simulink model "Pacemaker_A2_10_pushButton_bonus"  (R2020a)
settings: Solver=FixedStepAuto  StartTime=0.0  StopTime=10.0  FixedStep=1e-3  RelTol=1e-3  EnableMultiTasking=on
undefined symbols (not defined in the file): A0, A1, D0, D1, D10, D11, D12, D13, D2, D3, D4, D5, D6, D7, D8, D9, PTA0, PTA1, PTA2, PTB2, PTB23, PTB3, PTB9, PTC16, PTC17, PTC2, PTC3, PTC4, PTD0, PTD1, PTD2, PTD3
libraries: frdmk64flib x30, etargetslib x4
settings Model: ExtModeTrigDuration=5  Creator=forre  LastModifiedBy=forre
settings OptimizationCC: EnhancedBackFolding=on  PassReuseOutputArgsAs=Individual arguments  ZeroExternalMemoryAtStartup=off  ZeroInternalMemoryAtStartup=off  MaxStackSize=64  OptimizeBlockOrder=speed  DifferentSizesBufferReuse=on  OptimizationCustomize=off  EfficientTunableParamExpr=on
settings DebuggingCC: ParameterTunabilityLossMsg=error
settings HardwareCC: ProdBitPerPointer=32  ProdBitPerSizeT=32  ProdBitPerPtrDiffT=32  ProdLargestAtomicInteger=Long  ProdLargestAtomicFloat=Double  ProdWordSize=32  ProdHWDeviceType=ARM Compatible->ARM Cortex
settings SFSimCC: MATLABDynamicMemAlloc=off
settings RTWCC: SystemTargetFile=ert.tlc  HardwareBoard=NXP FRDM-K64F  TemplateMakefile=ert_default_tmf  Toolchain=GNU Tools for ARM Embedded Processors
settings CodeAppCC: ForceParamTrailComments=on  IgnoreCustomStorageClasses=off  OperatorAnnotations=on  SimulinkDataObjDesc=on  SFDataObjDesc=on  InsertBlockDesc=on

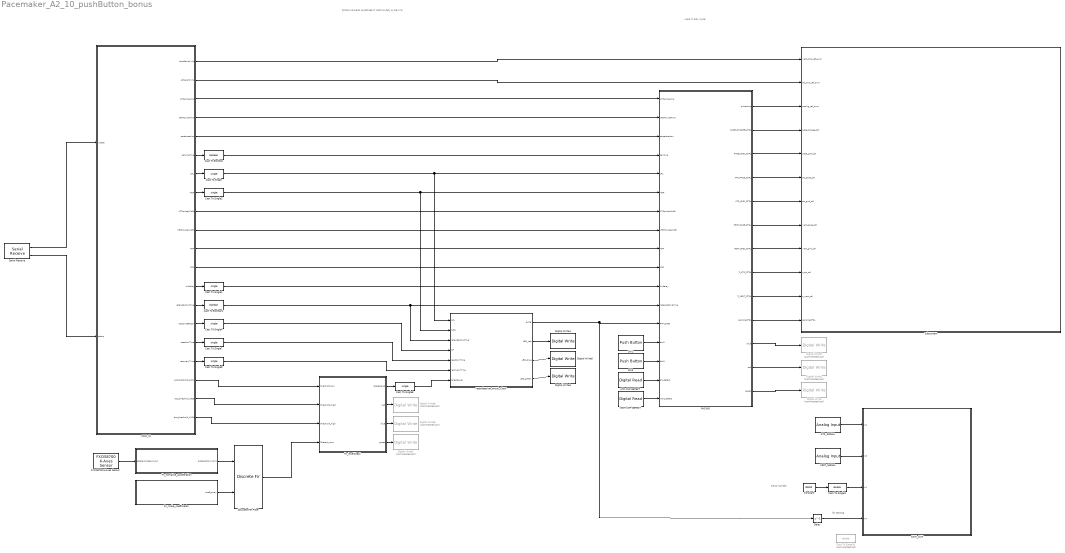
== system Pacemaker_A2_10_pushButton_bonus ==
  note: for testing
  note: serial number
  note: Python converts amplitude in Volts to duty cycle in %
  note: input = duty cycle
  ATR CMP DETECT : frdmk64flib/Digital Read  Whichpin=PTC16 (D0)  SampleTime=-1
  ATR_SIGNAL : frdmk64flib/Analog Input  Whichpin=PTB2 (A0)  SampleTime=0.01
  COM_IN : Stateflow chart  TreatAsAtomicUnit=on
      settings: PortSchema="{\"entries\":[{\"content\":{\"sides\":[{\"content\":{\"connectorIds\":[\"In1\",\"In2\"]},\"type\":\"ConnectorPlacement.EquallySpacedRectSide\",\"uuid\":\"708f6c47-59ba-4c62-823e-aceb534f7d4e\"},{\"content\":{\"connectorIds\":[\"Out1\",\"Out3\",\"Out2\",\"Out4\",\"Out5\",\"Out6\",\"Out7\",\"Out8\",\"Out9\",\"Out10\",\"Out11\",\"Out12\",\"Out13\",\"Out14\",\"Out15\",\"Out16\",\"Out17\",\"Out18\",\"Out19\",\"Out20\"],\"side\":\"RIGHT\"},\"type\":\"ConnectorPlacement.EquallySpacedRectSide\",\"uuid\":\"fc195095-7643-467f-bfab-06db9c9b4f5e\"},{\"content\":{\"connectorIds\":[],\"side\":\"TOP\"},\"type\":\"ConnectorPlacement.EquallySpacedRectSide\",\"uuid\":\"2b9dc66d-b3fc-4626-8ab6-5dc1815dc2f6\"}]},\"type\":\"ConnectorPlacement.EquallySpacedConnector\",\"uuid\":\"ad24e883-72a0-4c10-9901-797c84f459ab\"}],\"packageUris\":[\"http://schema.mathworks.com/mf0/Connector/19700101\"],\"version\":\"1.0\"}"
  COM_OUT : Subsystem
  Cast To Boolean : DataTypeConversion  OutDataTypeStr=boolean
  Cast To Boolean1 : DataTypeConversion  OutDataTypeStr=boolean
  Cast To Single{,1..2,4,7..9} (7 alike) : DataTypeConversion  OutDataTypeStr=single
  Cast To Single10 : DataTypeConversion  Commented=on  OutDataTypeStr=double
  Cast To Single3 : DataTypeConversion  OutDataTypeStr=double
  Constant : Constant  Value=92020
  Delay : Delay  DelayLength=1
  Digital Write : frdmk64flib/Digital Write  Commented=on  Whichpin=GREEN_LED
  Digital Write1 : frdmk64flib/Digital Write  Commented=on  Whichpin=RED_LED
  Digital Write2 : frdmk64flib/Digital Write  Commented=on  Whichpin=GREEN_LED
  Digital Write3 : frdmk64flib/Digital Write  Whichpin=GREEN_LED
  Digital Write4 : frdmk64flib/Digital Write  Whichpin=RED_LED
  Digital Write5 : frdmk64flib/Digital Write  Whichpin=BLUE_LED
  Digital Write6 : frdmk64flib/Digital Write  Commented=on  Whichpin=RED_LED
  Digital Write7 : frdmk64flib/Digital Write  Commented=on  Whichpin=BLUE_LED
  Digital Write8 : frdmk64flib/Digital Write  Commented=on  Whichpin=BLUE_LED
  Discrete FIR Filter : DiscreteFir  CoefSource=Input port  Coefficients=[0.05, 0.05, 0.05, 0.05, 0.05, 0.05, 0.05, 0.05, 0.05, 0.05, 0.05, 0.05, 0.05, 0.05, 0.05, 0.05, 0.05, 0.05, 0.05, 0.05]  SampleTime=0.01
      settings: InputPortMap=u0,u1
  FXOS8700 6-Axes Sensor : frdmk64flib/FXOS8700 6-Axes Sensor  Activesensor=Accelerometer only  ODR=800Hz  HybridODR=400Hz  Accelfullrange=-4g to +4g  SampleTime=-1
  Fn_levelCheck : MATLAB Function  TreatAsAtomicUnit=on
  Fn_make_coefficients : MATLAB Function  TreatAsAtomicUnit=on
  Fn_nomalize_acceleration : MATLAB Function  TreatAsAtomicUnit=on
  PACING : Stateflow chart  TreatAsAtomicUnit=on
  SW2 : frdmk64flib/Push Button  Whichswitch=SW2  SampleTime1=-1
  SW3 : frdmk64flib/Push Button  Whichswitch=SW3  SampleTime1=-1
  Serial Receive : frdmk64flib/Serial Receive  SCIModule=0  Baudrate=uint32(9600)  Parity=None  StopBits=1  HardwareFlowControl=None  ByteOrder=LittleEndian  DataType=uint8  DataLength=57  BlockingMode=off  OutputStatus=on  SampleTime=-1
  Subsystem : Subsystem
  VENT CMP DETECT : frdmk64flib/Digital Read  Whichpin=PTC17 (D1)  SampleTime=-1
  VENT_SIGNAL : frdmk64flib/Analog Input  Whichpin=PTB3 (A1)  SampleTime=0.01
  rateAdaptiveControl_Chart : Stateflow chart  TreatAsAtomicUnit=on
  wires:
  SW2/1 -> PACING/14(btn2)
  PACING/5(ATR_GND_CTRL) -> Subsystem/7(atr_gnd_ctrl)
  PACING/4(ATR_PACE_CTRL) -> Subsystem/6(atr_pace_ctrl)
  PACING/2(PACE_CHARGE_CTRL) -> Subsystem/4(pace_charge_ctrl)
  PACING/3(PACE_GND_CTRL) -> Subsystem/5(pace_gnd_ctrl)
  PACING/6(VENT_PACE_CTRL) -> Subsystem/8(vent_pace_ctrl)
  PACING/7(VENT_GND_CTRL) -> Subsystem/9(vent_gnd_ctrl)
  PACING/8(Z_ATR_CTRL) -> Subsystem/10(z_atr_ctrl)
  PACING/9(Z_VENT_CTRL) -> Subsystem/11(" z_vent_ctrl")
  ATR CMP DETECT/1 -> PACING/16(atr_detect)
  VENT CMP DETECT/1 -> PACING/17(vent_detect)
  PACING/10(sensingCTRL) -> Subsystem/12(sensingCTRL)
  COM_IN/6(sensingTrue) -> Cast To Boolean/1
  SW3/1 -> PACING/15(btn3)
  COM_IN/8(MSR) -> Cast To Single2/1
  COM_IN/11(ARP) -> PACING/9(ARP)
  COM_IN/12(VRP) -> PACING/10(VRP)
  Serial Receive/1 -> COM_IN/1(rxdata)
  Serial Receive/2 -> COM_IN/2(status)
  COM_IN/5(paceLocation) -> PACING/3(paceLocation)
  COM_IN/9(ATRpulseWidth) -> PACING/7(ATRpulseWidth)
  COM_IN/10(VENTpulseWidth) -> PACING/8(VENTpulseWidth)
  Cast To Boolean/1 -> PACING/4(sensing)
  COM_IN/7(LRL) -> Cast To Single/1
  PACING/1(pulseAmp) -> Subsystem/3(pacing_ref_pwm)
  COM_IN/1(VentSensitivity) -> Subsystem/1(vent_cmp_ref_pwm)
  COM_IN/3(AtrSensitivity) -> Subsystem/2(atr_cmp_ref_pwm)
  COM_IN/13(AVdelay) -> Cast To Single1/1
  Cast To Single3/1 -> COM_OUT/3(In1)
  VENT_SIGNAL/1 -> COM_OUT/2(In3)
  ATR_SIGNAL/1 -> COM_OUT/1(In2)
  Cast To Single1/1 -> PACING/11(AVdelay)
  PACING/11(blue) -> Digital Write7/1
  PACING/12(red) -> Digital Write1/1
  PACING/13(green) -> Digital Write/1
  COM_IN/2(ATRpulseAmp) -> PACING/1(ATRpulseAmp)
  COM_IN/4(VENTpulseAmp) -> PACING/2(VENTpulseAmp)
  rateAdaptiveControl_Chart/4(LED_green) -> Digital Write3/1
  Fn_nomalize_acceleration/1(acceleration_norm) -> Discrete FIR Filter/1
  Discrete FIR Filter/1 -> Fn_levelCheck/4(filtered_norm)
  Fn_make_coefficients/1(coeff_array) -> Discrete FIR Filter/2
  Fn_levelCheck/2(red) -> Digital Write6/1
  Fn_levelCheck/3(blue) -> Digital Write8/1
  Fn_levelCheck/1(targetLevel) -> Cast To Single8/1
  Fn_levelCheck/4(green) -> Digital Write2/1
  rateAdaptiveControl_Chart/2(LED_red) -> Digital Write4/1
  Cast To Single8/1 -> rateAdaptiveControl_Chart/7(targetLevel)
  rateAdaptiveControl_Chart/3(LED_blue) -> Digital Write5/1
  COM_IN/18(acc_threshold_LOW) -> Fn_levelCheck/1(threshold_low)
  COM_IN/19(acc_threshold_MED) -> Fn_levelCheck/2(threshold_med)
  COM_IN/20(acc_threshold_HIGH) -> Fn_levelCheck/3(threshold_high)
  COM_IN/15(responseFactor) -> Cast To Single4/1
  COM_IN/16(reactionTime) -> Cast To Single7/1
  COM_IN/17(recoveryTime) -> Cast To Single9/1
  Cast To Boolean1/1 -> rateAdaptiveControl_Chart/3(rateAdaptiveTrue), PACING/12(rateAdaptiveTrue)
  COM_IN/14(rateAdaptiveTrue) -> Cast To Boolean1/1
  Cast To Single/1 -> rateAdaptiveControl_Chart/1(LRL), PACING/5(LRL)
  Cast To Single2/1 -> rateAdaptiveControl_Chart/2(MSR), PACING/6(MSR)
  Cast To Single4/1 -> rateAdaptiveControl_Chart/4(RF)
  Cast To Single7/1 -> rateAdaptiveControl_Chart/5(reactionTime)
  Cast To Single9/1 -> rateAdaptiveControl_Chart/6(recoveryTime)
  Constant/1 -> Cast To Single3/1
  FXOS8700 6-Axes Sensor/1 -> Fn_nomalize_acceleration/1(accelerometer_input)
  Delay/1 -> COM_OUT/4(In4)
  rateAdaptiveControl_Chart/1(RATE) -> Delay/1, PACING/13(PPM_Rate)

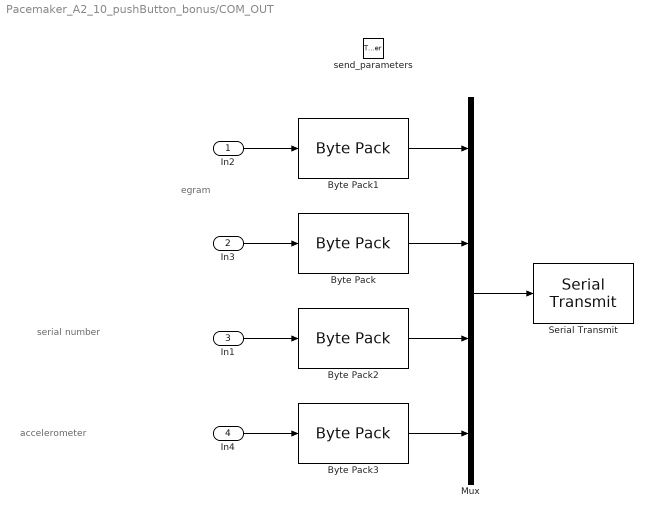
== system Pacemaker_A2_10_pushButton_bonus/COM_OUT ==
  note: egram
  note: accelerometer
  note: serial number
  In2 : Inport
  In3 : Inport  Port=2
  In1 : Inport  Port=3
  In4 : Inport  Port=4
  send_parameters : TriggerPort  TriggerType=function-call  IsSimulinkFunction=on  FunctionName=send_parameters  VariantControl=(inherit)
  Byte Pack : etargetslib/Byte Pack  datatypes={'double'}  byteAlign=1
  Byte Pack1 : etargetslib/Byte Pack  datatypes={'double'}  byteAlign=1
  Byte Pack2 : etargetslib/Byte Pack  datatypes={'double'}  byteAlign=1
  Byte Pack3 : etargetslib/Byte Pack  datatypes={'single'}  byteAlign=1
  Mux : Mux
  Serial Transmit : frdmk64flib/Serial Transmit  SCIModule=0  Baudrate=uint32(9600)  Parity=None  StopBits=1  HardwareFlowControl=None  ByteOrder=LittleEndian  BlockingMode=on  OutputStatus=off
  wires:
  Byte Pack/1 -> Mux/2
  Mux/1 -> Serial Transmit/1
  In3/1 -> Byte Pack/1
  In2/1 -> Byte Pack1/1
  Byte Pack1/1 -> Mux/1
  In1/1 -> Byte Pack2/1
  In4/1 -> Byte Pack3/1
  Byte Pack2/1 -> Mux/3
  Byte Pack3/1 -> Mux/4

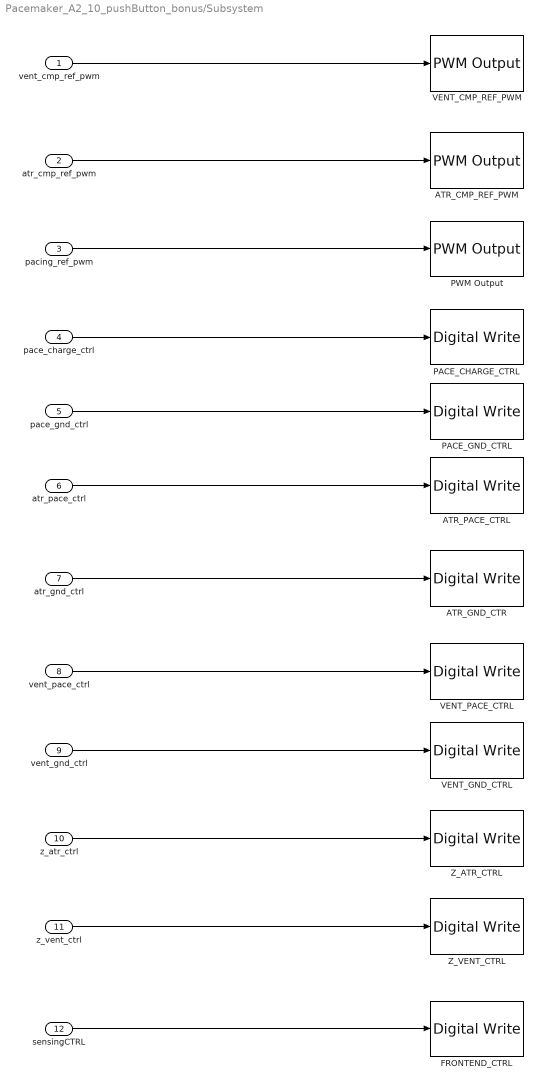
== system Pacemaker_A2_10_pushButton_bonus/Subsystem ==
  vent_cmp_ref_pwm : Inport
  atr_cmp_ref_pwm : Inport  Port=2
  pacing_ref_pwm : Inport  Port=3
  pace_charge_ctrl : Inport  Port=4
  pace_gnd_ctrl : Inport  Port=5
  atr_pace_ctrl : Inport  Port=6
  atr_gnd_ctrl : Inport  Port=7
  vent_pace_ctrl : Inport  Port=8
  vent_gnd_ctrl : Inport  Port=9
  z_atr_ctrl : Inport  Port=10
  " z_vent_ctrl" : Inport  Port=11
  sensingCTRL : Inport  Port=12
  ATR_CMP_REF_PWM : frdmk64flib/PWM Output  Whichpin=PTC2 (D6)  InitialFrequency=2000  InitialDutyCycle=50
  ATR_GND_CTR : frdmk64flib/Digital Write  Whichpin=PTD2 (D11)
  ATR_PACE_CTRL : frdmk64flib/Digital Write  Whichpin=PTA0 (D8)
  FRONTEND_CTRL : frdmk64flib/Digital Write  Whichpin=PTD1 (D13)
  PACE_CHARGE_CTRL : frdmk64flib/Digital Write  Whichpin=PTB9 (D2)
  PACE_GND_CTRL : frdmk64flib/Digital Write  Whichpin=PTD0 (D10)
  PWM Output : frdmk64flib/PWM Output  Whichpin=PTA2 (D5)  InitialFrequency=2000  InitialDutyCycle=50
  VENT_CMP_REF_PWM : frdmk64flib/PWM Output  Whichpin=PTA1 (D3)  InitialFrequency=2000  InitialDutyCycle=50
  VENT_GND_CTRL : frdmk64flib/Digital Write  Whichpin=PTD3 (D12)
  VENT_PACE_CTRL : frdmk64flib/Digital Write  Whichpin=PTC4 (D9)
  Z_ATR_CTRL : frdmk64flib/Digital Write  Whichpin=PTB23 (D4)
  Z_VENT_CTRL : frdmk64flib/Digital Write  Whichpin=PTC3 (D7)
  wires:
  pace_gnd_ctrl/1 -> PACE_GND_CTRL/1
  atr_pace_ctrl/1 -> ATR_PACE_CTRL/1
  pace_charge_ctrl/1 -> PACE_CHARGE_CTRL/1
  atr_gnd_ctrl/1 -> ATR_GND_CTR/1
  vent_pace_ctrl/1 -> VENT_PACE_CTRL/1
  vent_gnd_ctrl/1 -> VENT_GND_CTRL/1
  z_atr_ctrl/1 -> Z_ATR_CTRL/1
  " z_vent_ctrl"/1 -> Z_VENT_CTRL/1
  sensingCTRL/1 -> FRONTEND_CTRL/1
  pacing_ref_pwm/1 -> PWM Output/1
  vent_cmp_ref_pwm/1 -> VENT_CMP_REF_PWM/1
  atr_cmp_ref_pwm/1 -> ATR_CMP_REF_PWM/1

== stateflow chart Pacemaker_A2_10_pushButton_bonus/PACING ==
  note: beat sensed
  state SENSING_VENT_TRUE
    %sensing
  state VENT_CHARGING_AND_DISCHARGE
    entry:
    % for this state paceLocation = 1
    %begin charge and discharge cycle for ventricle
    msecPerPace = 60000.0/PPM_Rate; %new value in msec
    ATR_PACE_CTRL = false;
    VENT_PACE_CTRL = false;
    pulseAmp = VENTpulseAmp; % set amplitude
    PACE_CHARGE_CTRL = true;
    PACE_GND_CTRL = true;
    Z_VENT_CTRL = false;
    Z_ATR_CTRL = false
    VENT_GND_CTRL = true;
    ATR_GND_CTRL = false;
  note: switch to dual
  state VENT_PACING
    entry:
    % pace ventricle
    PACE_CHARGE_CTRL = false;
    PACE_GND_CTRL = true;
    VENT_PACE_CTRL = true;
    VENT_GND_CTRL = false;
    Z_VENT_CTRL = false;
    Z_ATR_CTRL = false;
    ATR_GND_CTRL = false;
    ATR_PACE_CTRL = false;
  note: VENT PACING
  note: bonus: inhibit pacing with button down
  note: switch to atr
  note: switch to vent
  state ATR_CHARGING_AND_DISCHARGE
    entry:
    % for this state paceLocation = 0
    %begin charge and discharge cycle for atrium
    msecPerPace = 60000.0/PPM_Rate; %new value for pace timing with msec units
    sensingCTRL = true; %enables the sensing circuitry if sensing = 1
    ATR_PACE_CTRL = false;
    VENT_PACE_CTRL = false;
    pulseAmp = ATRpulseAmp; % set amplitude
    PACE_CHARGE_CTRL = true;
    PACE_GND_CTRL = true;
    Z_VENT_CTRL = false;
    Z_ATR_CTRL = false;
    VENT_GND_CTRL = false;
    ATR_GND_CTRL = true;
    blue = false;
    red = false;
    green = false;
  state ATR_PACING
    entry:
    % pace atrium
    PACE_CHARGE_CTRL = false;
    PACE_GND_CTRL = true;
    VENT_PACE_CTRL = false;
    VENT_GND_CTRL = false;
    Z_VENT_CTRL = false;
    Z_ATR_CTRL = false;
    ATR_GND_CTRL = false;
    ATR_PACE_CTRL = true;
  note: switch to dual
  note: ATR PACING
  state SENSING_ATR_TRUE
    %sensing
  note: beat sensed
  state DUAL_SENSING_ATR_TRUE [commented out]
    %sensing
  note: beat sensed
  note: switch to atr
  state DUAL_ATR_CHARGING_AND_DISCHARGE_VENT
    entry:
    msecPerPace = 60000/PPM_Rate;
    % for this state paceLocation = 3
    %begin charge cycle for atrium
    ATR_PACE_CTRL = false;
    VENT_PACE_CTRL = false;
    pulseAmp = ATRpulseAmp; % set amplitude
    PACE_CHARGE_CTRL = true;
    PACE_GND_CTRL = true;
    Z_VENT_CTRL = false;
    Z_ATR_CTRL = false;
    VENT_GND_CTRL = true;
    ATR_GND_CTRL = false;
    blue = true;
    red = false;
    green = false;
  state DUAL_ATR_PACING
    entry:
    % pace atrium
    PACE_CHARGE_CTRL = false;
    PACE_GND_CTRL = true;
    VENT_PACE_CTRL = false;
    VENT_GND_CTRL = false;
    Z_VENT_CTRL = false;
    Z_ATR_CTRL = false;
    ATR_GND_CTRL = false;
    ATR_PACE_CTRL = true;
  note: switch to vent
  note: pace ATR
  note: DUAL PACING
  state DUAL_DISCHARGE_ATR_AND_VENT_CHARGING
    entry:
    %begin charge cycle for VENT
    ATR_PACE_CTRL = false;
    VENT_PACE_CTRL = false;
    pulseAmp = VENTpulseAmp;
    PACE_CHARGE_CTRL = true;
    PACE_GND_CTRL = true;
    Z_VENT_CTRL = false;
    Z_ATR_CTRL = false
    VENT_GND_CTRL = false;
    ATR_GND_CTRL = true;
    green = true;
  note: pace VENT
  state DUAL_VENT_PACING
    entry:
    % pace ventricle
    ATR_GND_CTRL = false;
    ATR_PACE_CTRL = false;
    PACE_CHARGE_CTRL = false;
    PACE_GND_CTRL = true;
    VENT_PACE_CTRL = true;
    VENT_GND_CTRL = false;
    Z_VENT_CTRL = false;
    Z_ATR_CTRL = false;
    red = true;
  note: bonus: inhibit pacing with button down
  state INHIBIT
    entry:
    if btn2
    inhibit = true;
    else
    inhibit = false;
    end
  VENT_CHARGING_AND_DISCHARGE -> SENSING_VENT_TRUE [order 2] : after((VRP-VENTpulseWidth),msec)[sensing && (vent_detect || btn3)]
  SENSING_VENT_TRUE -> VENT_CHARGING_AND_DISCHARGE : after(VENTpulseWidth, msec)
  VENT_CHARGING_AND_DISCHARGE -> DUAL_ATR_CHARGING_AND_DISCHARGE_VENT [order 4] : [paceLocation==3]
  VENT_PACING -> VENT_CHARGING_AND_DISCHARGE : after(VENTpulseWidth, msec)
  VENT_CHARGING_AND_DISCHARGE -> VENT_PACING [order 1] : after((msecPerPace-VENTpulseWidth), msec)
  DUAL_ATR_CHARGING_AND_DISCHARGE_VENT -> VENT_CHARGING_AND_DISCHARGE [order 2] : [paceLocation==2]
  ATR_CHARGING_AND_DISCHARGE -> VENT_CHARGING_AND_DISCHARGE [order 3] : [paceLocation==2]
  VENT_CHARGING_AND_DISCHARGE -> VENT_CHARGING_AND_DISCHARGE [order 5] : [btn2]
  VENT_CHARGING_AND_DISCHARGE -> ATR_CHARGING_AND_DISCHARGE [order 3] : [paceLocation==1]
  ATR_PACING -> ATR_CHARGING_AND_DISCHARGE : after(ATRpulseWidth, msec)
  (default) -> ATR_CHARGING_AND_DISCHARGE
  ATR_CHARGING_AND_DISCHARGE -> ATR_PACING [order 1] : after((msecPerPace-ATRpulseWidth), msec)
  ATR_CHARGING_AND_DISCHARGE -> DUAL_ATR_CHARGING_AND_DISCHARGE_VENT [order 4] : [paceLocation==3]
  DUAL_ATR_CHARGING_AND_DISCHARGE_VENT -> ATR_CHARGING_AND_DISCHARGE [order 1] : [paceLocation==1]
  ATR_CHARGING_AND_DISCHARGE -> SENSING_ATR_TRUE [order 2] : after((ARP-ATRpulseWidth),msec)[sensing && (atr_detect || btn3)]
  SENSING_ATR_TRUE -> ATR_CHARGING_AND_DISCHARGE : after(ATRpulseWidth, msec)
  DUAL_ATR_CHARGING_AND_DISCHARGE_VENT -> DUAL_SENSING_ATR_TRUE [commented out] : after((ARP-ATRpulseWidth),msec)[sensing && (atr_detect)]
  DUAL_SENSING_ATR_TRUE -> DUAL_ATR_CHARGING_AND_DISCHARGE_VENT [commented out] : after(ATRpulseWidth, msec)
  INHIBIT -> DUAL_ATR_PACING [order 2] : after(msecPerPace-AVdelay,msec)
  DUAL_ATR_CHARGING_AND_DISCHARGE_VENT -> DUAL_ATR_PACING [order 3] : after(msecPerPace-VENTpulseWidth-AVdelay,msec)
  DUAL_ATR_PACING -> DUAL_DISCHARGE_ATR_AND_VENT_CHARGING : after(ATRpulseWidth,msec)
  DUAL_VENT_PACING -> DUAL_ATR_CHARGING_AND_DISCHARGE_VENT : after(VENTpulseWidth,msec)
  DUAL_DISCHARGE_ATR_AND_VENT_CHARGING -> INHIBIT : after(AVdelay-ATRpulseWidth,msec)
  INHIBIT -> DUAL_VENT_PACING [order 1] : [~inhibit]
  data: pulseAmp output single; ATRpulseAmp input single; VENTpulseAmp input single; paceLocation input uint8; sensing input boolean; LRL input single; MSR input single; ATRpulseWidth input single; VENTpulseWidth input single; ARP input single; VRP input single; AVdelay input single; rateAdaptiveTrue input boolean; PPM_Rate input single; PACE_CHARGE_CTRL output boolean; PACE_GND_CTRL output boolean; btn2 input boolean; btn3 input boolean; ATR_PACE_CTRL output boolean; ATR_GND_CTRL output boolean; msecPerBeat local single; VENT_PACE_CTRL output boolean; VENT_GND_CTRL output boolean; Z_ATR_CTRL output boolean; Z_VENT_CTRL output boolean; atr_detect input boolean; vent_detect input boolean; sensingCTRL output boolean; msecPerPace local single; blue output boolean; red output boolean; green output boolean; inhibit local boolean
  data paceLocation settings: description=|
      | 0 = pace atrium
      | 1 = pace ventricle
  data atr_detect settings: description=|
      | 0 = pace atrium
      | 1 = pace ventricle
  data vent_detect settings: description=|
      | 0 = pace atrium
      | 1 = pace ventricle

== stateflow chart Pacemaker_A2_10_pushButton_bonus/rateAdaptiveControl_Chart ==
  state INITIALIZE
    entry:
    previousLevel = 0;
    RATE=LRL;
  note: if level = 0
      | RATE = LRL
      |
      | if level = 1
      | RATE = LRL + ResponseFactor
      |
      | if level = 2
      | RATE = LRL + 2*ResponseFactor
      |
      | if level = 3
      | RATE = LRL + 3*ResponseFactor
  state START
    entry:
    reactionTime_remaining = reactionTime;
    recoveryTime_remaining = recoveryTime;
    LED_red = false;
    LED_blue = false;
    LED_green = true;
    during:
    if ~rateAdaptiveTrue
    RATE = LRL;
    end
  note: incrementTime=reactionTime/((TargetLevel - PreviousLevel)*RF)
  note: IF target level < previous level
  note: decrease
  note: IF target level > previous level
  note: Increase
  state INCREMENT
    entry:
    incrementTime=reactionTime/((target - previousLevel)*RF);
    % time/BPM increase
    LED_green = false;
    if RATE < LRL
    RATE = LRL;
    elseif RATE > MSR
    RATE = MSR;
    end
  state DECREMENT
    entry:
    decrementTime=recoveryTime/((previousLevel - target)*RF);
    % time/BPM increase
    LED_green = false;
    if RATE < LRL
    RATE = LRL;
    elseif RATE > MSR
    RATE = MSR;
    end
  note: [reactionTime_remaining>0]
  (default) -> INITIALIZE
  INITIALIZE -> START
  START -> START [commented out] : [~rateAdaptiveTrue]{RATE = LRL;}
  START -> INCREMENT [order 1] : [targetLevel > previousLevel && rateAdaptiveTrue]{target = targetLevel}
  START -> DECREMENT [order 2] : [targetLevel < previousLevel && rateAdaptiveTrue]{target = targetLevel}
  INCREMENT -> START [order 1] : [(reactionTime_remaining <= 0) || (targetLevel <= previousLevel) || ~rateAdaptiveTrue]{previousLevel = target}
  DECREMENT -> START [order 1] : [(recoveryTime_remaining <= 0) || (targetLevel >= previousLevel) || ~rateAdaptiveTrue]{previousLevel = target}
  INCREMENT -> INCREMENT [order 2] : after(incrementTime,sec){RATE=RATE+1;reactionTime_remaining=reactionTime_remaining-incrementTime;LED_blue = true;}
  DECREMENT -> DECREMENT [order 2] : after(decrementTime, sec)[recoveryTime_remaining>0]{RATE=RATE-1;recoveryTime_remaining=recoveryTime_remaining-decrementTime;LED_red = true;}
  data: LRL input single; MSR input single; rateAdaptiveTrue input boolean; RF input single; reactionTime input single; RATE output single; previousLevel local single; recoveryTime input single; decrementTime local single; incrementTime local single; reactionTime_remaining local single; recoveryTime_remaining local single; targetLevel input single; LED_red output boolean; LED_blue output boolean; target local single; LED_green output boolean

== stateflow chart Pacemaker_A2_10_pushButton_bonus/COM_IN ==
  state SET_PARAMETERS
    entry:
    paceLocation = rxdata(3); %1 if ATRIUM, 2 if VENT, 3 if BOTH
    sensingTrue = rxdata(4); %1 if sensing, 0 if not
    LRL = rxdata(5);
    MSR =  rxdata(6);
    ATRpulseAmp = typecast(rxdata(7:10), 'single');
    VENTpulseAmp = typecast(rxdata(11:14),'single');
    ATRpulseWidth = typecast(rxdata(15:18),'single');
    VENTpulseWidth = typecast(rxdata(19:22),'single');
    ARP = typecast(rxdata(23:26),'single');
    VRP = typecast(rxdata(27:30),'single');
    AtrSensitivity = typecast(rxdata(31:34), 'single');
    VentSensitivity = typecast(rxdata(35:38), 'single');
    AVdelay = typecast(rxdata(39:40), 'uint16');
    rateAdaptiveTrue =  typecast(rxdata(41),'uint8');
    responseFactor = typecast(rxdata(42),'uint8');
    acc_threshold_LOW = typecast(rxdata(43:46), 'single');
    acc_threshold_MED = typecast(rxdata(47:50), 'single');
    acc_threshold_HIGH = typecast(rxdata(51:54), 'single');
    reactionTime = typecast(rxdata(55),'uint8');
    recoveryTime = typecast(rxdata(56:57), 'uint16');
  state INITIAL
    entry:
    paceLocation = 1; %1 if atr, 2 if vent, 3 if dual
    sensingTrue = 0; %1 if sensing, 0 if not
    LRL = 60; %ppm
    MSR = 120; %ppm
    ATRpulseAmp = 50; %duty cycle
    VENTpulseAmp = 50; %duty cycle
    ATRpulseWidth = 10; %msec
    VENTpulseWidth = 10; %msec
    ARP = 250; %msec
    VRP = 250; %msec
    AtrSensitivity = 50; %duty cycle
    VentSensitivity = 50; %duty cycle
    AVdelay = 50.0; %msec
    rateAdaptiveTrue = 0; %uint
    acc_threshold_LOW = 1.1; %ajust according to Accelerometer single
    acc_threshold_MED = 1.5;
    acc_threshold_HIGH = 2;
    responseFactor = 1; % 1-16
    reactionTime = 10; % sec uint8
    recoveryTime = 30; % sec uint16
  note: receive values
  state STANDBY
    %waiting
  note: send values
  state ECHO_PARAMETERS
    entry:
    send_parameters();
  SET_PARAMETERS -> STANDBY
  (default) -> INITIAL
  (junction 14) -> SET_PARAMETERS [order 1] : [rxdata(2) == hex2dec('55')]
  (junction 18) -> STANDBY [order 2]
  INITIAL -> STANDBY
  STANDBY -> (junction 18) : [status==0]
  (junction 18) -> (junction 14) [order 1] : [rxdata(1) == hex2dec('16')]
  (junction 14) -> ECHO_PARAMETERS [order 2] : [rxdata(2) == hex2dec('22')]
  ECHO_PARAMETERS -> STANDBY
  data: VentSensitivity output single; ATRpulseAmp output single; AtrSensitivity output single; VENTpulseAmp output single; paceLocation output uint8; sensingTrue output uint8; LRL output uint8; MSR output uint8; ATRpulseWidth output single; VENTpulseWidth output single; ARP output single; rxdata input uint8; VRP output single; status input uint8; AVdelay output uint16; rateAdaptiveTrue output uint8; responseFactor output uint8; reactionTime output uint8; recoveryTime output uint16; acc_threshold_LOW output single; acc_threshold_MED output single; acc_threshold_HIGH output single

== matlab function Pacemaker_A2_10_pushButton_bonus/Fn_nomalize_acceleration ==
  data: accelerometer_input input; acceleration_norm output
function acceleration_norm = fcn(accelerometer_input)
acceleration_norm = sqrt((accelerometer_input(1))^2+(accelerometer_input(2))^2+(accelerometer_input(3))^2);

== matlab function Pacemaker_A2_10_pushButton_bonus/Fn_levelCheck ==
  data: targetLevel output; threshold_low input; threshold_med input; threshold_high input; filtered_norm input; red output; blue output; green output
function [targetLevel, red, blue, green] = fcn(threshold_low,threshold_med,threshold_high, filtered_norm)
red = false;
blue = false;
green = false;

if filtered_norm >= threshold_high
    targetLevel = 3;
    red = true;

elseif filtered_norm >= threshold_med
    targetLevel = 2;
    green = true;
    
elseif filtered_norm >= threshold_low
    targetLevel = 1;
    blue = true;
    
else
    targetLevel = 0;
    
    red = false;
    blue = false;
    green = false;
end

== matlab function Pacemaker_A2_10_pushButton_bonus/Fn_make_coefficients ==
  data: coeff_array output double
function coeff_array = fcn()
coeff_array= ones(500,1)/500;
